simulink model "Lista2"  (R2023b)
settings: Solver=FixedStepAuto  StartTime=0.0  StopTime=10  FixedStep=0.0001  MaxStep=0.0001  MinStep=0.0001  RelTol=1e-3
settings Model: Creator=solem  LastModifiedBy=solem
settings SolverCC: InitialStep=0.0001

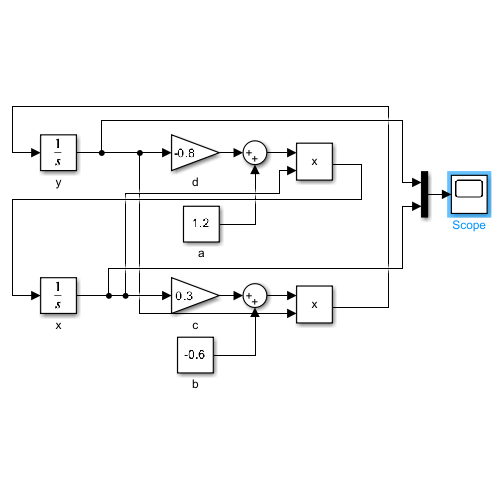
[thumbnail: Simulink's stored preview of the top-level diagram]
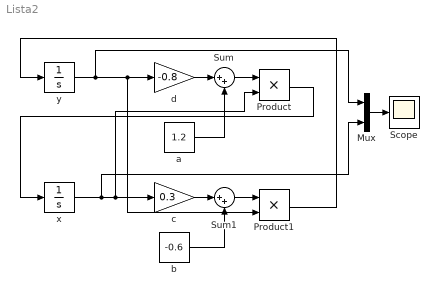
== system Lista2 ==
  Mux : Mux  Inputs=2
  Product : Product
  Product1 : Product
  Scope : Scope
  Sum : Sum  Inputs=|++
  Sum1 : Sum  Inputs=|++
  a : Constant  Value=1.2
  b : Constant  Value=-0.6
  c : Gain  Gain=0.3
  d : Gain  Gain=-0.8
  x : Integrator  InitialCondition=2
  y : Integrator  InitialCondition=1
  wires:
  y/1 -> Mux/1, Product1/2, d/1
  d/1 -> Sum/1
  a/1 -> Sum/2
  x/1 -> Mux/2, c/1, Product/2
  c/1 -> Sum1/1
  b/1 -> Sum1/2
  Sum/1 -> Product/1
  Sum1/1 -> Product1/1
  Product1/1 -> y/1
  Product/1 -> x/1
  Mux/1 -> Scope/1
